simulink library "FindUnitVectorComponents_ul"  (R2018a)
settings: Solver=VariableStepAuto  StartTime=0.0  StopTime=10.0  RelTol=1e-3
settings Model: Creator=mcobb  LastModifiedBy=mcobb

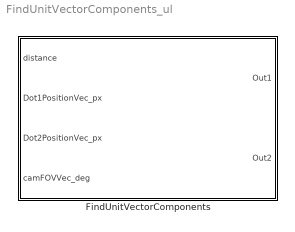
== system FindUnitVectorComponents_ul ==
  FindUnitVectorComponents : Subsystem

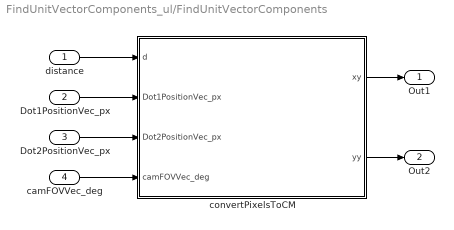
== system FindUnitVectorComponents_ul/FindUnitVectorComponents ==
  distance : Inport
  Dot1PositionVec_px : Inport  Port=2
  Dot2PositionVec_px : Inport  Port=3
  camFOVVec_deg : Inport  Port=4  PortDimensions=2
  convertPixelsToCM : MATLAB Function  TreatAsAtomicUnit=on
  Out1 : Outport
  Out2 : Outport  Port=2
  wires:
  convertPixelsToCM/1(xy) -> Out1/1
  convertPixelsToCM/2(yy) -> Out2/1
  distance/1 -> convertPixelsToCM/1(d)
  camFOVVec_deg/1 -> convertPixelsToCM/4(camFOVVec_deg)
  Dot1PositionVec_px/1 -> convertPixelsToCM/2(Dot1PositionVec_px)
  Dot2PositionVec_px/1 -> convertPixelsToCM/3(Dot2PositionVec_px)

== matlab function FindUnitVectorComponents_ul/FindUnitVectorComponents/convertPixelsToCM ==
  data: d input; xy output size=1; yy output size=1; Dot1PositionVec_px input; Dot2PositionVec_px input; camFOVVec_deg input
function [xy, yy] = ...
    convertPixelsToLength(d,Dot1PositionVec_px,Dot2PositionVec_px,camFOVVec_deg)
%#codegen

% INPUTS:
% d - distance from camera to dot centroid
% xLeft - horizontal pixel coordinate location of left dot in the frame
% xRight - horizontal pixel coordinate location of the right dot in the
% frame
% yLeft - vertical pixel coordinate location of the left dot in the frame
% yRight -  vertical pixel coordinate location of the right dot in the
% frame
% viewAngle - two element vector, first characterizes the width of the
% field of view (camera horizontal), the second characterizes the height of
% the field of veiw (camera vertical).
xLeft = Dot1PositionVec_px(2);
yLeft = Dot1PositionVec_px(1);

xRight = Dot2PositionVec_px(2);
yRight = Dot2PositionVec_px(1);

% Calculate dot separations in pixels
% Camera-X separation will contribute to y component of body fixed y unit
% vector, if left dot is to the left of right dot (xLeft<xRight), then the 
% component will have a positive value.  Camera-Y separation
% will contribute to x component of body fixed y unit vector if left dot is
% below right dot (yLeft>yRight),
% then this should have a positive value.
yy = -(xLeft - xRight); 
xy =  (yLeft - yRight);

% Convert pixels to length
% The (2*d*tand(viewAngle(1))) term calculates the total horizontal (or
% vertical)
% distance spanned by the camera field of view, the /2040 and /1080 terms
% normalize the separations by the total number of pixels.
xy = (2*d*tand(camFOVVec_deg(1)))*(xy/2040); % y component of body fixed y
yy = (2*d*tand(camFOVVec_deg(2)))*(yy/1080); % z component of body fixed y


yc=(xLeft+xRight)/2;
xc=(yLeft+yRight)/2;
yy = yy/cosd(20*((544-yc)/544));
xy = xy/cosd(20*((1020-xc)/1020));
